simulink model "Lab4_Minimize_Transmission_Loss_in_Power_Sys_with_Transf"  (R2024b)
settings: Solver=VariableStepAuto  StartTime=0.0  StopTime=10.0  RelTol=1e-3
undefined symbols (not defined in the file): Angle, Magnitude
libraries: spsCurrentMeasurementLib x4, spsSeriesRLCBranchLib x4, spsACVoltageSourceLib x2, spsLinearTransformerLib x2, spsVoltageMeasurementLib x2, sps_lib x1
settings Model: Creator=DELL  LastModifiedBy=DELL

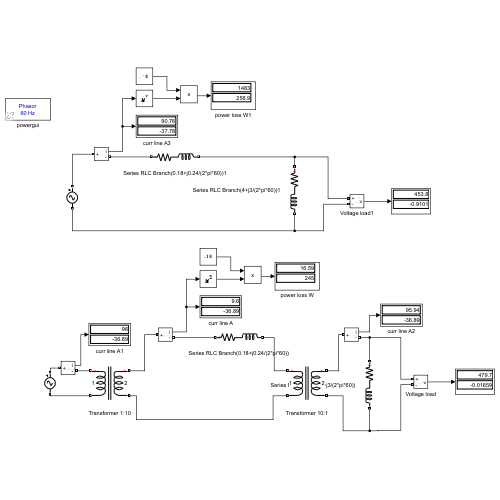
[thumbnail: Simulink's stored preview of the top-level diagram]
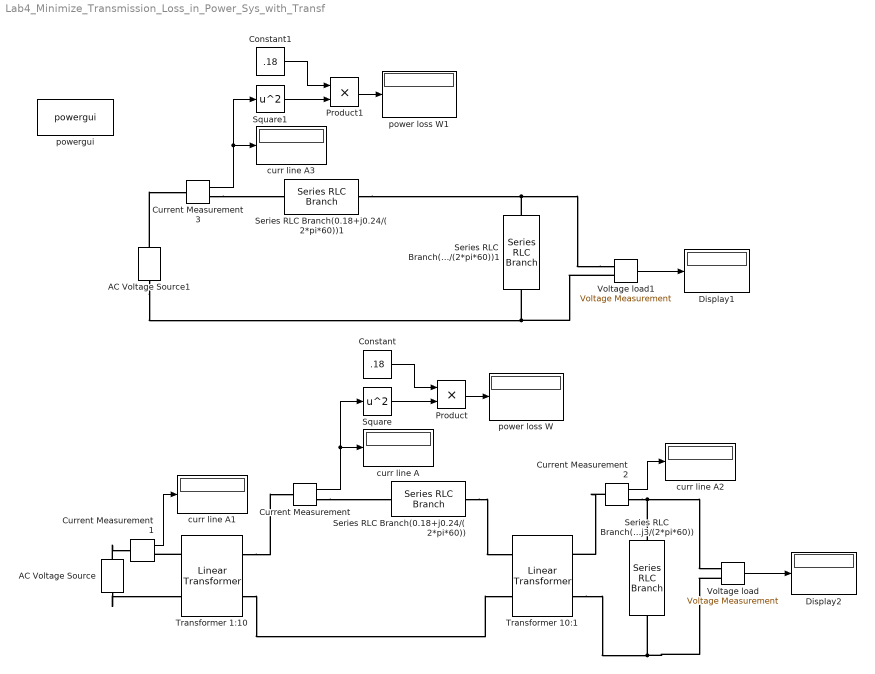
== system Lab4_Minimize_Transmission_Loss_in_Power_Sys_with_Transf ==
  AC Voltage Source : spsACVoltageSourceLib/AC Voltage Source  Amplitude=480  Phase=0  Frequency=60  SampleTime=0  Measurements=None  BusType=swing  Pref=10e3  Qref=0  Qmin=-inf  Qmax=+inf
  AC Voltage Source1 : spsACVoltageSourceLib/AC Voltage Source  Amplitude=480  Phase=0  Frequency=60  SampleTime=0  Measurements=None  BusType=swing  Pref=10e3  Qref=0  Qmin=-inf  Qmax=+inf
  Constant : Constant  Value=.18
  Constant1 : Constant  Value=.18
  Current Measurement{,1..3} (4 alike) : spsCurrentMeasurementLib/Current Measurement  PhasorSimulation=on  OutputType=Magnitude-Angle  PSBequivalent=0
  Display1 : Display
  Display2 : Display
  Product : Product
  Product1 : Product
  Series RLC Branch(0.18+j0.24/(2*pi*60)) : spsSeriesRLCBranchLib/Series RLC Branch  LConnTagsString=__new0  RConnTagsString=__new0  BranchType=RL  Resistance=0.18  Inductance=0.24/(2*pi*60)  SetiL0=off  InitialCurrent=0  Capacitance=1e-6  Setx0=off  InitialVoltage=0  Measurements=None
  Series RLC Branch(0.18+j0.24/(2*pi*60))1 : spsSeriesRLCBranchLib/Series RLC Branch  LConnTagsString=__new0  RConnTagsString=__new0  BranchType=RL  Resistance=0.18  Inductance=0.24/(2*pi*60)  SetiL0=off  InitialCurrent=0  Capacitance=1e-6  Setx0=off  InitialVoltage=0  Measurements=None
  Series RLC Branch(4+j3/(2*pi*60)) : spsSeriesRLCBranchLib/Series RLC Branch  LConnTagsString=__new0  RConnTagsString=__new0  BranchType=RL  Resistance=4  Inductance=3/(2*pi*60)  SetiL0=off  InitialCurrent=0  Capacitance=1e-6  Setx0=off  InitialVoltage=0  Measurements=None
  Series RLC Branch(4+j3/(2*pi*60))1 : spsSeriesRLCBranchLib/Series RLC Branch  LConnTagsString=__new0  RConnTagsString=__new0  BranchType=RL  Resistance=4  Inductance=3/(2*pi*60)  SetiL0=off  InitialCurrent=0  Capacitance=1e-6  Setx0=off  InitialVoltage=0  Measurements=None
  Square : Math  Operator=square
  Square1 : Math  Operator=square
  Transformer 10:1 : spsLinearTransformerLib/Linear Transformer  UNITS=SI  NominalPower=[ 250e6 60 ]  winding1=[4800 0.000001 0.000001]  winding2=[480 0.000001 0.000001]  ThreeWindings=off  winding3=[3.15e+05 0.7938 0.084225]  RmLm=[1.0804e+06 2866]  Measurements=None  DataType=on
  Transformer 1:10 : spsLinearTransformerLib/Linear Transformer  UNITS=SI  NominalPower=[ 250e6 60 ]  winding1=[480 0.000001 0.000001]  winding2=[4800 0.000001 0.000001]  ThreeWindings=off  winding3=[3.15e+05 0.7938 0.084225]  RmLm=[1.0804e+06 2866]  Measurements=None  DataType=on
  Voltage load : spsVoltageMeasurementLib/Voltage Measurement  PhasorSimulation=on  OutputType=Magnitude-Angle  PSBequivalent=0
  Voltage load1 : spsVoltageMeasurementLib/Voltage Measurement  PhasorSimulation=on  OutputType=Magnitude-Angle  PSBequivalent=0
  curr line A{,1..3} (4 alike) : Display
  power loss W : Display
  power loss W1 : Display
  powergui : sps_lib/powergui  Priority=1  SimulationMode=Phasor  SampleTime=50e-6  frequency=60  Iterations=50  frequencyindice=60  Pbase=100e6  ErrMax=1e-4  UnitsV=kV  UnitsW=MW  buscounter=0  FunctionMessages=off  echomessages=off  EnableUseOfTLC=off  CurrentSourceSwitches=off  DisableSnubberDevices=off  DisableRonSwitches=off  DisableVfSwitches=off  DisplayEquations=off  AutomaticDiscreteSolvers=off  SolverType=Tustin/Backward Euler (TBE)  Interpol=off  ExternalGateDelay=off  methode=off  Ts=100  x0status=blocks  SPID=on  SwTol=0  HookPort=off  NonlinearTolerance=1e-4  nMaxIteration=100  ContinueOnMaxIteration=off  RestoreLinks=warning  ResistiveCurrentMeasurement=off  Frange=[0:2:500]  Ylog=off  Xlog=on  ShowGrid=off  save=off  variable=ZData  structure=0  ZoomFFT=off  StartTime=0.0  cycles=1  DisplayStyle=1  fundamental=60  FreqAxis=off  MaxFrequency=1000  frequencyindicesteady=1  RmsSteady=1  display=off
  wires:
  Current Measurement/1 -> Square/1, curr line A/1
  Square/1 -> Product/2
  Constant/1 -> Product/1
  Product/1 -> power loss W/1
  Voltage load/1 -> Display2/1
  Current Measurement1/1 -> curr line A1/1
  Current Measurement2/1 -> curr line A2/1
  Voltage load1/1 -> Display1/1
  Constant1/1 -> Product1/1
  Product1/1 -> power loss W1/1
  Square1/1 -> Product1/2
  Current Measurement3/1 -> Square1/1, curr line A3/1
  connections:
  Series RLC Branch(4+j3/(2*pi*60))/LConn1 -- Current Measurement2/RConn1 -- Voltage load/LConn1
  Voltage load/LConn2 -- Transformer 10:1/RConn2 -- Series RLC Branch(4+j3/(2*pi*60))/RConn1
  Current Measurement/RConn1 -- Series RLC Branch(0.18+j0.24/(2*pi*60))/LConn1
  AC Voltage Source/RConn1 -- Current Measurement1/LConn1
  Transformer 1:10/LConn1 -- Current Measurement1/RConn1
  AC Voltage Source/LConn1 -- Transformer 1:10/LConn2
  Series RLC Branch(0.18+j0.24/(2*pi*60))/RConn1 -- Transformer 10:1/LConn1
  Transformer 1:10/RConn2 -- Transformer 10:1/LConn2
  Transformer 1:10/RConn1 -- Current Measurement/LConn1
  Current Measurement2/LConn1 -- Transformer 10:1/RConn1
  Voltage load1/LConn1 -- Series RLC Branch(0.18+j0.24/(2*pi*60))1/RConn1 -- Series RLC Branch(4+j3/(2*pi*60))1/LConn1
  Current Measurement3/RConn1 -- Series RLC Branch(0.18+j0.24/(2*pi*60))1/LConn1
  AC Voltage Source1/RConn1 -- Current Measurement3/LConn1
  AC Voltage Source1/LConn1 -- Voltage load1/LConn2 -- Series RLC Branch(4+j3/(2*pi*60))1/RConn1
